simulink model "Expriment_All2"  (R2014a)
settings: Solver=FixedStepDiscrete  SolverMode=SingleTasking  StartTime=0.0  StopTime=inf  FixedStep=0.01  RelTol=1e-3
PostLoadFcn:
  | h_RPStest = RPStest;
model workspace (MAT data in the model file):
  gtest = 0
undefined symbols (not defined in the file or in its folder): avert, avert_freq_factor, avert_gaze_dirs_chance, avert_gaze_duration_factor, avert_head_frequency_factor, avert_head_speed, BML, BML1, BML2, bmlsL, bmlsM, bodyBusyFlag, clock, emotion_amount_factor, faceBusyFlag, fileID, GAZE_WIN, gazing, mut_freq_factor, mutual_gaze_duration_factor, P, pose_cat_chance, pose_chanc_factor, pose_chance_factor, pose_frequency_factor, pose_lean, pose_lean_flag, pose_speed, pose_twitch, pr, serial, STATE_BEFORE, STATE_GO, STATE_OVER, STATE_READY, Stateflow
libraries: simulink x24, instrumentlib x6, lib_affectiveChar_behavior x2, realtime_pacer_lib x2, lib_affectiveChar_input x1
(part 7 of 7)

== stateflow chart Expriment_All2/CharacterControl/Gaze_Controller ==
  note: ?
  note: ?
  note: implement PERSONALITY-based gaze behavior: ( setAffectFactors function)
      | HEHN:mutual dur more,head avert freq more,high freq of change btw mut/avert
      | LEHN:avert dur  more,head avert freq more, high freq of change btw mut/avert
      | HELN:mutual dur  more,head avert freq more,high freq of change btw mut/avert
      | LELN:avert  dur more,head avert freq more,high freq of change btw mut/avert
  note: ?
  note: implement emotion-based gaze behavior, Valence/Arousal: ref?(setAffectFactors)
      | V+A+ (excite,happy):high mutual dur,head avert freq less,high freq of change btw mut/avert
      | V-A+ (fear,frust): mid mut/avert,,head avert freq mid,high freq of change btw mut/avert
      | V+A- (idle, calm): mid mut/avert,head avert freq mid,low freq of change btw mut/avert
      | V-A- (bored,sad):  avert dur more,,head avert freq more,,high freq of change btw mut/avert
  note: Idle gaze impelementation:
      | For chanceO instead of range btw 5,15 we pick 3,15; 3,8 for eye due to Smartbody gaze DOF(5', 12') and 9 to 15 for head
      | A=saccade magnitude
      | CHANCEO=P=chance of occure (random num btw 0 and 15)  -> for us:3 to 8
      | magnitude=A=-6.9 * log(P/15.7), A is a value btw 0 and 27 ->for us: 5 to 12
      | Eye Alives' Image 5
      | -Saccade direction: Up/Down/Left/Right/UL/UR/DL/DR
      | 15% chance of pures and 8% chance of others.
      | -Duration D=D0+d*A-> avertDur=(25+2.5*magnitude)->36 to 52
      | d=2.4 msec/degree;  D0=25
      | For more info check Badler's Eye's Alive paper
  note: Idle gaze impelementation cont.:
      |
      | mut=Percent chance of stay in mutual gaze based on time is mut=[0.0003 -0.18 32]  %chance of no change from mutual =Y=0.0003x2 - 0.18 x +32
      | polyval(mut,t) %  t btw 1 to 400, mut btw 30 and 4
      |
      | avert=Percent chance of stay in avert gaze based on time:   avert=[-0.0034 0.23 -6.7 79]
      | polyval(avert,t)  % t btw 0 and 60 , avert btw 79 and -100?!
      | Eye's Alive paper's image 7
  note: avert_head_frequency_factor:
      | Riggio suggested that extraverts have a higher head movement frequency than introverts.
      | Riggio, R., Friedman, H. 1986. Impression formation: The role of expressive behavior. In Journal of Personality and Social Psychology 50(2), 421-427
  note: impelemnt attention:
      | all gaze movements are based on gazeTarget pawn in smartbody. Idle gaze stops when agent attends something since it gazes that. If user starts moving the idle gaze stops.It also stops in RPS game,ready and go states.
  note: Extroverts maintain eye-contact for longer.
      | Mehrabian, A. 1969. Significance of posture and position in
      | the communication of attitude and status relationships. In
      | Psychological Bulletin 71(5), 359-372.
  note: Note on modulization of affect (personality/emotion): I could have a seperate module for affect impact on all behaviors (gaze/pose/face). But I see the personality not as a seperate module but as a factor on (or layer on top of) eachbehavior. That's why I defined a matlab function (affect) in which emotion/personality facors affects different parameters of each behavior inside that behavior module. But for modulization, I also specify 0 as no personality in case someone don't want to use it.
  state headAvert [parallel]
    settings: executionOrder=2
    state stateInit1
      entry: STATE_OVER=3;STATE_BEFORE=4;STATE_READY=7;STATE_GO=1; gameState=14;
      GAZE_GUI=1;GAZE_SOFTEYE=2;GAZE_USER_HAND=3;GAZE_WIN=4;
      n=encStr2Arr(' ');bmlsL=[n n n n n];newBmlsL=[n n n n n];
      avert_head_speed=1;avertH=0;
    state stateRandGen1
      entry:
      gazeUserHandChance=randArray(:,4);gazeGUIChance=randArray(:,5);
      randHeadDur=((25+2.5*magnitude)*avert_gaze_duration_factor)/3;
    state stateHeadNeutralN1
      entry: [P,BMLl]= idleNormalHeadTable(12);
      newBmlsL=insertQueueLow(bmlsL,BMLl); bmlsL=newBmlsL;
      avertH=0;
    state stateAvertHeadNormal
      entry: avert=1; [P,BMLl]= idleNormalHeadTable(randArray(:,18));
      newBmlsL=insertQueueLow(bmlsL,BMLl); bmlsL=newBmlsL;
    state stateHeadNeutralF1
      entry: [P,BMLl]= idleFastUpHeadTable(22) ;
      newBmlsL=insertQueueLow(bmlsL,BMLl); bmlsL=newBmlsL;
      avertH=0;
    state stateAvertHeadFast%btw(1,20)
      entry: avert=1; [P,BMLl]= idleFastUpHeadTable(randArray(:,18));
      newBmlsL=insertQueueLow(bmlsL,BMLl); bmlsL=newBmlsL;
      %disp(decArr2Str(BMLl));
    state stateHeadNeutralS1
      entry: [P,BMLl]= idleSlowDownHeadTable(19) ;
      newBmlsL=insertQueueLow(bmlsL,BMLl); bmlsL=newBmlsL;
      avertH=0;
    state stateAvertHeadSlow%btw(1,18)
      entry: avert=1; [P,BMLl]= idleSlowDownHeadTable(randArray(:,19));
      newBmlsL=insertQueueLow(bmlsL,BMLl); bmlsL=newBmlsL;
    state stateGazingGUI
      entry: [P,BMLl]=  idleGazeTable(22) ;
      newBmlsL=insertQueueLow(bmlsL,BMLl); bmlsL=newBmlsL;
    state stateGazingUserHand
      entry: [P,BMLl]= idleGazeTable(23);
      newBmlsL=insertQueueLow(bmlsL,BMLl); bmlsL=newBmlsL;
    (default) -> stateInit1
    stateInit1 -> stateRandGen1 : [avertH==1]
    stateRandGen1 -> stateRandGen1 [order 4] : after(floor(randHeadDur/5),secs)
    stateRandGen1 -> stateGazingUserHand [order 2] : [([gazeUserHandChance==1])&([gazing==GAZE_USER_HAND])]
    stateRandGen1 -> stateGazingGUI [order 3] : [([gazeGUIChance==1])&([gazing==GAZE_GUI])]
    stateRandGen1 -> (junction 539) [order 1] : [[bodyBusyFlag~=1]&[faceBusyFlag~=1]&[ gameState~= STATE_GO]&[ gameState~= STATE_READY]&[avertH==1]]
    stateHeadNeutralS1 -> stateRandGen1 : after(2,secs)
    stateHeadNeutralF1 -> stateRandGen1 : after(2,secs)
    stateHeadNeutralN1 -> stateRandGen1 : after(2,secs)
    (junction 539) -> stateAvertHeadNormal [order 2] : [avert_head_speed==1]
    (junction 539) -> stateAvertHeadFast%btw(1,20) [order 1] : [avert_head_speed==2]
    (junction 539) -> stateAvertHeadSlow%btw(1,18) [order 3] : [avert_head_speed==3]
    stateAvertHeadNormal -> stateHeadNeutralN1 : after(randHeadDur,secs)
    (junction 508) -> stateHeadNeutralN1 [order 2] : [avert_head_speed==1]
    stateAvertHeadFast%btw(1,20) -> stateHeadNeutralF1 : after(randHeadDur,secs)
    (junction 508) -> stateHeadNeutralF1 [order 1] : [avert_head_speed==2]
    stateAvertHeadSlow%btw(1,18) -> stateHeadNeutralS1 : after(randHeadDur+20,secs)
    (junction 508) -> stateHeadNeutralS1 [order 3] : [avert_head_speed==3]
    stateGazingGUI -> (junction 508) : after(10,secs)
    stateGazingUserHand -> (junction 508) : after(10,secs)
  state stateGazeIde [parallel]
    settings: executionOrder=1
    state setBlinkRate
      entry: str= blinkFunction(blinkperiod_min,blinkperiod_max) ;
      sendSBM(str);blink_flag=0;
    state stateInit
      entry: STATE_OVER=3;STATE_BEFORE=4;STATE_READY=7;STATE_GO=1; gameState=14;
      n=encStr2Arr(' ');bmlsL=[n n n n n];newBmlsL=[n n n n n];
      mutual_gaze_duration_factor=1;avert_gaze_duration_factor=1;avert_gaze_dirs_chance=0;
      avert_freq_factor=1;mut_freq_factor=1;avert_head_frequency_factor=20;
      avert=1;avertH=0;currentTime=1;
      blink_flag=0;blinkperiod_min=5;blinkperiod_max=9;
    note: if already mutual do not send mut bml.
    state mutAgain
      entry:chanceO=randArray(:,17);
      magnitude=-6.9*log(chanceO/15.7);
      mutDur=((25+2.5*magnitude)*mutual_gaze_duration_factor)/7;
    state stateCheckMutCont
      entry:  coder.extrinsic('get_param');
      currentTime=get_param('Expriment_All','SimulationTime');
      mutContF=[0.0003 -0.18 32];
      CHANCEM=randArray(:,6);%btw 0,100
      mutContChance=polyval(mutContF,currentTime);
      mutContChance=mutContChance*mut_freq_factor;
    state stateAvert
      entry:%btw 1,100
      randHeadChance=randArray(:,3);
    state stateAvertEye
      entry:  avert=1;
      chanceO=randArray(:,7);%btw 3,8
      magnitude=-6.9*log(chanceO/15.7);
      avertDur=((25+2.5*magnitude)*avert_gaze_duration_factor)/7;
      gazeDir=randArray(:,8);
      BMLl= idleGazeFunction(gazeDir,floor(magnitude),avert_gaze_dirs_chance) ;
      newBmlsL=insertQueueLow(bmlsL,BMLl);
      bmlsL=newBmlsL;%fprintf(',A:'); fprintf('%1.1f',avertDur);
    state stateAvertHead
      entry:avertH=1;
      chanceH=randArray(:,25);%btw 8,15
      magnitude=-6.9*log(chanceH/15.7);
      avertDur=((25+2.5*magnitude)*avert_gaze_duration_factor)/7;
      gazeDir=randArray(:,8);
    state stateMutualGazeE
      entry:chanceO=randArray(:,17);%btw 3,8
      magnitude=-6.9*log(chanceO/15.7);
      mutDur=((25+2.5*magnitude)*mutual_gaze_duration_factor)/7;
      [P,BMLl]= idleNormalHeadTable(11) ;%neutralGaze
      avert=0;
      newBmlsL=insertQueueLow(bmlsL,BMLl);
      bmlsL=newBmlsL;%fprintf(',M:'); fprintf('%1.1f',mutDur);
    state stateCheckAvertCont
      entry:
      coder.extrinsic('get_param');
      currentTime=get_param('Expriment_All','SimulationTime');
      %avertContF=[-0.0034 0.23 -6.7 79];
      avertContF=[0.0003 -0.18 32];
      avertContChance=polyval(avertContF,currentTime);
      avertContChance=avertContChance*avert_freq_factor;
      CHANCEA=randArray(:,9);%btw 0,100
    setBlinkRate -> stateAvert [order 2]
    stateAvert -> setBlinkRate [order 1] : [blink_flag==1]%order first
    stateCheckMutCont -> setBlinkRate [order 1] : [blink_flag==1]%order first
    setBlinkRate -> stateCheckMutCont [order 1] : after(5,secs)
    (default) -> stateInit
    stateInit -> stateCheckMutCont : [[bodyBusyFlag~=1]&[faceBusyFlag~=1]&[ gameState~= STATE_GO]&[ gameState~= STATE_READY]]
    mutAgain -> stateCheckMutCont : after(floor(mutDur),secs)
    stateCheckMutCont -> mutAgain [order 4] : [avert==0]%order after avert 1
    stateAvert -> (junction 577) [order 2]
    (junction 577) -> stateAvertEye [order 1] : [avert_head_frequency_factor<=randHeadChance]
    (junction 577) -> stateAvertHead [order 2] : [avert_head_frequency_factor>randHeadChance]
    stateCheckMutCont -> stateAvert [order 2] : [[CHANCEM>mutContChance]&[bodyBusyFlag~=1]&[faceBusyFlag~=1]&[ gameState~= STATE_GO]&[ gameState~= STATE_READY]]
    (junction 200) -> stateAvert [order 2] : [[CHANCEA<=avertContChance]&[ gameState~= STATE_GO]&[ gameState~= STATE_READY]]
    stateCheckMutCont -> (junction 323) [order 3] : [[avert==1]&[CHANCEM<=mutContChance]&[bodyBusyFlag~=1]&[faceBusyFlag~=1]&[ gameState~= STATE_GO]&[ gameState~= STATE_READY]]
    stateMutualGazeE -> stateCheckMutCont : after(floor(mutDur),secs)
    stateAvertHead -> (junction 588) : [avertH==0]
    stateAvertEye -> (junction 581) : after(floor(avertDur),secs)
    (junction 588) -> (junction 581) : after(5,secs)
    (junction 581) -> stateCheckAvertCont
    stateCheckAvertCont -> (junction 200)
    (junction 200) -> (junction 323) [order 1] : [[avertH==0]&[CHANCEA>avertContChance]&[ gameState~= STATE_GO]&[ gameState~= STATE_READY]]
    (junction 323) -> stateMutualGazeE
  note: idleGaze(1,8) used for gaze,
      | idleGaze(9,16) used for head,
      | idleGaze(17) used for neutralHead
      | idleGaze(18) used for gaze at board
  note: The result of facial expr module showed that if we only consider emotion on facial expr generation, it leads to non-consistent behavior because emotion also affects how we gaze, pose and gesture. If your face shows boredom but there is no evidence in other parts of the body it looks not consistent.
      | But the question is how much of these behaviors are affected by personality and how much with emotion. e.g. highly extroverts seems to mutual gaze more, is it because they generally experience more positive valence. or neurotics avert more is it becasue of high arousal?
  state sendSBM(In) [function]
  data: p function_output double size=1; bmlID function_input double; gazeBML function_output double size=[1000,1]; p function_output double size=1; bmlID function_input double; gazeBML function_output double size=[1000,1]; p function_output double size=1; bmlID function_input double; gazeBML function_output double size=[1000,1]; p function_output double size=1; bmlID function_input double; gazeBML function_output double size=[1000,1]; p function_output double size=1; bmlID function_input double size=1; gazeBML function_output double size=[1000,1]; p function_output double size=1; bmlID function_input double; gazeBML function_output double size=[1000,1]; dir function_input double size=1; mag function_input double size=1; arrBML function_output double size=[1000,1]; p function_output double size=1; bmlID function_input double; poseBML function_output double size=[1000,1]; dir function_input double size=1; mag function_input double size=1; arrBML function_output double size=[1000,1]; dirChance function_input double size=1; headSpeed function_input double size=1; dir function_input double size=1; mag function_input double size=1; arrBML function_output double size=[1000,1]; dirChance function_input double size=1; bmls function_input double size=[1000,5]; myBML function_input double size=[1000,1]; newBmls function_output double size=[1000,5]; blinkPeriodMin function_input double size=1; arrSBM function_output double size=[1000,1]; blinkPeriodMax function_input double size=1; In function_input double size=[1000 1]; boredom data_store_memory size=2; BOREDOM_THRESHOLD data_store_memory size=2; randAvertGazeChance data_store_memory size=2; randPoseChance data_store_memory size=2; interest data_store_memory size=2; randGazeDur data_store_memory size=2; gazing data_store_memory size=2; GAZE_SOFTEYE data_store_memory size=2; GAZE_GUI data_store_memory size=2; GAZE_USER_HAND data_store_memory size=2; GAZE_WIN data_store_memory size=2; randHeadDur local; randHeadDurOver local; gameState output double size=1; avert data_store_memory size=2; STATE_BEFORE data_store_memory size=2; STATE_OVER data_store_memory size=2; STATE_READY data_store_memory size=2; avertContChance local; gazeGUIChance local; mutContChance local; mutContF local; CHANCEM local; avertDur local; gazeDir local; CHANCEA local; magnitude local; randHeadChance local; avertContF local; gazeUserHandChance local; bmlsL data_store_memory size=[256,1]; pr data_store_memory; P data_store_memory; chanceO local; fileID data_store_memory; STATE_GO data_store_memory; bodyBusyFlag data_store_memory; BMLl local double size=[1000,1]; BML data_store_memory size=[256,1]; newBmlsL local double size=[1000,5]; n local; randArray input double size=[1,40]; mutDur local; personality input double size=1; mF local; hF local; aF local; avertH data_store_memory; inV input double size=1; inA input size=1; mFe local; hFe local; aFe local; personalityChange input boolean size=1; faceBusyFlag data_store_memory; gazeArray input double size=[1,6]; avert_gaze_dirs_chance data_store_memory; avert_head_speed data_store_memory; avert_head_frequency_factor data_store_memory; avert_gaze_duration_factor data_store_memory; mutual_gaze_duration_factor data_store_memory; chanceH local; currentTime local; avert_freq_factor data_store_memory; mut_freq_factor data_store_memory; blink_flag data_store_memory; blinkperiod_min data_store_memory; str local; blinkperiod_max data_store_memory
  events: secs input RISING_EDGE_EVENT
  function [p,gazeBML]=idleSlowDownHeadTable(bmlID):
    | function [p,gazeBML]=idleSlowDownHeadTable(bmlID)
    | 
    | aVarTruthTableCondition_1 = false;
    | aVarTruthTableCondition_2 = false;
    | aVarTruthTableCondition_3 = false;
    | aVarTruthTableCondition_4 = false;
    | aVarTruthTableCondition_5 = false;
    | aVarTruthTableCondition_6 = false;
    | aVarTruthTableCondition_7 = false;
    | aVarTruthTableCondition_8 = false;
    | aVarTruthTableCondition_9 = false;
    | aVarTruthTableCondition_10 = false;
    | aVarTruthTableCondition_11 = false;
    | aVarTruthTableCondition_12 = false;
    | aVarTruthTableCondition_13 = false;
    | aVarTruthTableCondition_14 = false;
    | aVarTruthTableCondition_15 = false;
    | aVarTruthTableCondition_16 = false;
    | aVarTruthTableCondition_17 = false;
    | aVarTruthTableCondition_18 = false;
    | aVarTruthTableCondition_19 = false;
    | 
    | 
    | 
    | aVarTruthTableCondition_1 = logical(bmlID==1);
    | 
    | 
    | aVarTruthTableCondition_2 = logical(bmlID==2);
    | 
    | 
    | aVarTruthTableCondition_3 = logical(bmlID==3);
    | 
    | 
    | aVarTruthTableCondition_4 = logical(bmlID==4);
    | 
    | 
    | aVarTruthTableCondition_5 = logical(bmlID==5);
    | 
    | 
    | aVarTruthTableCondition_6 = logical(bmlID==6);
    | 
    | 
    | aVarTruthTableCondition_7 = logical(bmlID==7);
    | 
    | 
    | aVarTruthTableCondition_8 = logical(bmlID==8);
    | 
    | 
    | aVarTruthTableCondition_9 = logical(bmlID==9);
    | 
    | 
    | aVarTruthTableCondition_10 = logical(bmlID==10);
    | 
    | 
    | aVarTruthTableCondition_11 = logical(bmlID==11);
    | 
    | 
    | aVarTruthTableCondition_12 = logical(bmlID==12);
    | 
    | 
    | aVarTruthTableCondition_13 = logical(bmlID==13);
    | 
    | 
    | aVarTruthTableCondition_14 = logical(bmlID==14);
    | 
    | 
    | aVarTruthTableCondition_15 = logical(bmlID==15);
    | 
    | 
    | aVarTruthTableCondition_16 = logical(bmlID==16);
    | 
    | 
    | aVarTruthTableCondition_17 = logical(bmlID==17);
    | 
    | 
    | aVarTruthTableCondition_18 = logical(bmlID==18);
    | 
    | 
    | aVarTruthTableCondition_19 = logical(bmlID==19);
    | 
    | if (aVarTruthTableCondition_1)
    |     aFcnTruthTableAction_1();
    | elseif (aVarTruthTableCondition_2)
    |     aFcnTruthTableAction_2();
    | elseif (aVarTruthTableCondition_3)
    |     aFcnTruthTableAction_3();
    | elseif (aVarTruthTableCondition_4)
    |     aFcnTruthTableAction_4();
    | elseif (aVarTruthTableCondition_5)
    |     aFcnTruthTableAction_1();
    | elseif (aVarTruthTableCondition_6)
    |     aFcnTruthTableAction_2();
    | elseif (aVarTruthTableCondition_7)
    |     aFcnTruthTableAction_3();
    | elseif (aVarTruthTableCondition_8)
    |     aFcnTruthTableAction_4();
    | elseif (aVarTruthTableCondition_9)
    |     aFcnTruthTableAction_5();
    | elseif (aVarTruthTableCondition_10)
    |     aFcnTruthTableAction_6();
    | elseif (aVarTruthTableCondition_11)
    |     aFcnTruthTableAction_7();
    | elseif (aVarTruthTableCondition_12)
    |     aFcnTruthTableAction_8();
    | elseif (aVarTruthTableCondition_13)
    |     aFcnTruthTableAction_9();
    | elseif (aVarTruthTableCondition_14)
    |     aFcnTruthTableAction_10();
    | elseif (aVarTruthTableCondition_15)
    |     aFcnTruthTableAction_11();
    | elseif (aVarTruthTableCondition_16)
    |     aFcnTruthTableAction_12();
    | elseif (aVarTruthTableCondition_17)
    |     aFcnTruthTableAction_13();
    | elseif (aVarTruthTableCondition_18)
    |     aFcnTruthTableAction_14();
    | elseif (aVarTruthTableCondition_19)
    |     aFcnTruthTableAction_15();
    | else % Default
    |     aFcnTruthTableAction_1();
    | end
    | 
    | function aFcnTruthTableAction_1()
    | 
    | % DownleftHeadSlow1
    | 
    | gazeBML=encStr2Arr('<?xml version="1.0" ?><act><bml><gaze direction="DOWNLEFT" angle="15" sbm:joint-range="EYES NECK" sbm:time-hint="1.2" target="gazeTarget"/></bml></act>');p=3;
    | 
    | function aFcnTruthTableAction_2()
    | 
    | % DownleftHeadSlow2
    | 
    | gazeBML=encStr2Arr('<?xml version="1.0" ?><act><bml><gaze direction="DOWNLEFT" angle="20" sbm:joint-range="EYES NECK" sbm:time-hint="1.2" target="gazeTarget"/></bml></act>');p=3;
    | 
    | function aFcnTruthTableAction_3()
    | 
    | % DownleftHeadSlow3
    | 
    | gazeBML=encStr2Arr('<?xml version="1.0" ?><act><bml><gaze direction="DOWNLEFT" angle="25" sbm:joint-range="EYES NECK" sbm:time-hint="1.2" target="gazeTarget"/></bml></act>');p=3;
    | 
    | function aFcnTruthTableAction_4()
    | 
    | % DownleftHeadSlow4
    | 
    | gazeBML=encStr2Arr('<?xml version="1.0" ?><act><bml><gaze direction="DOWNLEFT" angle="30" sbm:joint-range="EYES NECK" sbm:time-hint="1.2" target="gazeTarget"/></bml></act>');p=3;
    | 
    | function aFcnTruthTableAction_5()
    | 
    | % DownrightHeadSlow1
    | 
    | gazeBML=encStr2Arr('<?xml version="1.0" ?><act><bml><gaze direction="DOWNRIGHT" angle="15" sbm:joint-range="EYES NECK" sbm:time-hint="1.2" target="gazeTarget"/></bml></act>');p=3;
    | 
    | function aFcnTruthTableAction_6()
    | 
    | % DownrightHeadSlow2
    | 
    | gazeBML=encStr2Arr('<?xml version="1.0" ?><act><bml><gaze direction="DOWNRIGHT" angle="20" sbm:joint-range="EYES NECK" sbm:time-hint="1.2" target="gazeTarget"/></bml></act>');p=3;
    | 
    | function aFcnTruthTableAction_7()
    | 
    | % DownrightHeadSlow3
    | 
    | gazeBML=encStr2Arr('<?xml version="1.0" ?><act><bml><gaze direction="DOWNRIGHT" angle="25" sbm:joint-range="EYES NECK" sbm:time-hint="1.2" target="gazeTarget"/></bml></act>');p=3;
    | 
    | function aFcnTruthTableAction_8()
    | 
    | % DownrightHeadSlow4
    | 
    | gazeBML=encStr2Arr('<?xml version="1.0" ?><act><bml><gaze direction="DOWNRIGHT" angle="30" sbm:joint-range="EYES NECK" sbm:time-hint="1.2" target="gazeTarget"/></bml></act>');p=3;
    | 
    | function aFcnTruthTableAction_9()
    | 
    | % DownHeadSlow1
    | 
    | gazeBML=encStr2Arr('<?xml version="1.0" ?><act><bml><gaze direction="DOWN" angle="15" sbm:joint-range="EYES NECK" sbm:time-hint="1.2" target="gazeTarget"/></bml></act>');p=3;
    | 
    | function aFcnTruthTableAction_10()
    | 
    | % DownHeadSlow2
    | 
    | gazeBML=encStr2Arr('<?xml version="1.0" ?><act><bml><gaze direction="DOWN" angle="20" sbm:joint-range="EYES NECK" sbm:time-hint="1.2" target="gazeTarget"/></bml></act>');p=3;
    | 
    | function aFcnTruthTableAction_11()
    | 
    | % DownHeadSlow3
    | 
    | gazeBML=encStr2Arr('<?xml version="1.0" ?><act><bml><gaze direction="DOWN" angle="25" sbm:joint-range="EYES NECK" sbm:time-hint="1.2" target="gazeTarget"/></bml></act>');p=3;
    | 
    | function aFcnTruthTableAction_12()
    | 
    | % DownHeadSlow4
    | 
    | gazeBML=encStr2Arr('<?xml version="1.0" ?><act><bml><gaze direction="DOWN" angle="30" sbm:joint-range="EYES NECK" sbm:time-hint="1.2" target="gazeTarget"/></bml></act>');p=3;
    | 
    | function aFcnTruthTableAction_13()
    | 
    | % LEFTHeadDSlow
    | 
    | gazeBML=encStr2Arr('<?xml version="1.0" ?><act><bml><gaze direction="DOWNLEFT" angle="10" sbm:joint-range="EYES NECK" sbm:time-hint="1.2" target="gazeTarget"/></bml></act>');p=3;
    | 
    | function aFcnTruthTableAction_14()
    | 
    | % RightHeadDSlow
    | 
    | gazeBML=encStr2Arr('<?xml version="1.0" ?><act><bml><gaze direction="DOWNRIGHT" angle="10" sbm:joint-range="EYES NECK" sbm:time-hint="1.2" target="gazeTarget"/></bml></act>');p=3;
    | 
    | function aFcnTruthTableAction_15()
    | 
    | % introvertHeadNeutral
    | 
    | gazeBML=encStr2Arr('<?xml version="1.0" ?><act><bml><gaze angle="5" direction="DOWN" sbm:joint-range="EYES BACK" sbm:time-hint="1.2" target="gazeTarget"/></bml></act>'); p=3;
  function [p,gazeBML]=idleGazeTable(bmlID):
    | function [p,gazeBML]=idleGazeTable(bmlID)
    | 
    | aVarTruthTableCondition_1 = false;
    | aVarTruthTableCondition_2 = false;
    | aVarTruthTableCondition_3 = false;
    | aVarTruthTableCondition_4 = false;
    | aVarTruthTableCondition_5 = false;
    | aVarTruthTableCondition_6 = false;
    | aVarTruthTableCondition_7 = false;
    | aVarTruthTableCondition_8 = false;
    | aVarTruthTableCondition_9 = false;
    | aVarTruthTableCondition_10 = false;
    | aVarTruthTableCondition_11 = false;
    | aVarTruthTableCondition_12 = false;
    | aVarTruthTableCondition_13 = false;
    | aVarTruthTableCondition_14 = false;
    | aVarTruthTableCondition_15 = false;
    | aVarTruthTableCondition_16 = false;
    | aVarTruthTableCondition_17 = false;
    | aVarTruthTableCondition_18 = false;
    | aVarTruthTableCondition_19 = false;
    | aVarTruthTableCondition_20 = false;
    | aVarTruthTableCondition_21 = false;
    | aVarTruthTableCondition_22 = false;
    | aVarTruthTableCondition_23 = false;
    | 
    | 
    | 
    | aVarTruthTableCondition_1 = logical(bmlID==1);
    | 
    | 
    | aVarTruthTableCondition_2 = logical(bmlID==2);
    | 
    | 
    | aVarTruthTableCondition_3 = logical(bmlID==3);
    | 
    | 
    | aVarTruthTableCondition_4 = logical(bmlID==4);
    | 
    | 
    | aVarTruthTableCondition_5 = logical(bmlID==5);
    | 
    | 
    | aVarTruthTableCondition_6 = logical(bmlID==6);
    | 
    | 
    | aVarTruthTableCondition_7 = logical(bmlID==7);
    | 
    | 
    | aVarTruthTableCondition_8 = logical(bmlID==8);
    | 
    | 
    | aVarTruthTableCondition_9 = logical(bmlID==9);
    | 
    | 
    | aVarTruthTableCondition_10 = logical(bmlID==10);
    | 
    | 
    | aVarTruthTableCondition_11 = logical(bmlID==11);
    | 
    | 
    | aVarTruthTableCondition_12 = logical(bmlID==12);
    | 
    | 
    | aVarTruthTableCondition_13 = logical(bmlID==13);
    | 
    | 
    | aVarTruthTableCondition_14 = logical(bmlID==14);
    | 
    | 
    | aVarTruthTableCondition_15 = logical(bmlID==15);
    | 
    | 
    | aVarTruthTableCondition_16 = logical(bmlID==16);
    | 
    | % neutralHead
    | 
    | aVarTruthTableCondition_17 = logical(bmlID==17);
    | 
    | % gazeAtGUIRachel
    | 
    | aVarTruthTableCondition_18 = logical(bmlID==18);
    | 
    | % softeye
    | 
    | aVarTruthTableCondition_19 = logical(bmlID==19);
    | 
    | % softeyebrow
    | 
    | aVarTruthTableCondition_20 = logical(bmlID==20);
    | 
    | % gazeUserHand
    | 
    | aVarTruthTableCondition_21 = logical(bmlID==21);
    | 
    | % gazeGUIBrad
    | 
    | aVarTruthTableCondition_22 = logical(bmlID==22);
    | 
    | % gazeHandBrad
    | 
    | aVarTruthTableCondition_23 = logical(bmlID==23);
    | 
    | if (aVarTruthTableCondition_1)
    |     aFcnTruthTableAction_1();
    | elseif (aVarTruthTableCondition_2)
    |     aFcnTruthTableAction_2();
    | elseif (aVarTruthTableCondition_3)
    |     aFcnTruthTableAction_3();
    | elseif (aVarTruthTableCondition_4)
    |     aFcnTruthTableAction_4();
    | elseif (aVarTruthTableCondition_5)
    |     aFcnTruthTableAction_5();
    | elseif (aVarTruthTableCondition_6)
    |     aFcnTruthTableAction_6();
    | elseif (aVarTruthTableCondition_7)
    |     aFcnTruthTableAction_7();
    | elseif (aVarTruthTableCondition_8)
    |     aFcnTruthTableAction_8();
    | elseif (aVarTruthTableCondition_9)
    |     aFcnTruthTableAction_9();
    | elseif (aVarTruthTableCondition_10)
    |     aFcnTruthTableAction_10();
    | elseif (aVarTruthTableCondition_11)
    |     aFcnTruthTableAction_11();
    | elseif (aVarTruthTableCondition_12)
    |     aFcnTruthTableAction_12();
    | elseif (aVarTruthTableCondition_13)
    |     aFcnTruthTableAction_13();
    | elseif (aVarTruthTableCondition_14)
    |     aFcnTruthTableAction_14();
    | elseif (aVarTruthTableCondition_15)
    |     aFcnTruthTableAction_15();
    | elseif (aVarTruthTableCondition_16)
    |     aFcnTruthTableAction_16();
    | elseif (aVarTruthTableCondition_17)
    |     aFcnTruthTableAction_17();
    | elseif (aVarTruthTableCondition_18)
    |     aFcnTruthTableAction_18();
    | elseif (aVarTruthTableCondition_19)
    |     aFcnTruthTableAction_19();
    | elseif (aVarTruthTableCondition_20)
    |     aFcnTruthTableAction_20();
    | elseif (aVarTruthTableCondition_21)
    |     aFcnTruthTableAction_21();
    | elseif (aVarTruthTableCondition_22)
    |     aFcnTruthTableAction_22();
    | elseif (aVarTruthTableCondition_23)
    |     aFcnTruthTableAction_23();
    | else % Default
    |     aFcnTruthTableAction_1();
    | end
    | 
    | function aFcnTruthTableAction_1()
    | 
    | % LeftS
    | 
    | gazeBML=encStr2Arr('<?xml version="1.0" ?><act><bml><gaze angle="12" direction="LEFT" sbm:joint-range="EYES" target="gazeTarget"/></bml></act>');p=3;
    | 
    | function aFcnTruthTableAction_2()
    | 
    | % RightS
    | 
    | gazeBML=encStr2Arr('<?xml version="1.0" ?><act><bml><gaze angle="12" direction="RIGHT" sbm:joint-range="EYES" target="gazeTarget"/></bml></act>');p=3;
    | 
    | function aFcnTruthTableAction_3()
    | 
    | % UpS
    | 
    | gazeBML=encStr2Arr('<?xml version="1.0" ?><act><bml><gaze angle="12" direction="UP" sbm:joint-range="EYES" target="gazeTarget"/></bml></act>');p=3;
    | 
    | function aFcnTruthTableAction_4()
    | 
    | % DownS
    | 
    | gazeBML=encStr2Arr('<?xml version="1.0" ?><act><bml><gaze angle="12" direction="DOWN" sbm:joint-range="EYES" target="gazeTarget"/></bml></act>');p=3;
    | 
    | function aFcnTruthTableAction_5()
    | 
    | % UpLeftS
    | 
    | gazeBML=encStr2Arr('<?xml version="1.0" ?><act><bml><gaze angle="12" direction="UPLEFT" sbm:joint-range="EYES" target="gazeTarget"/></bml></act>');p=3;
    | 
    | function aFcnTruthTableAction_6()
    | 
    | % UpRightS
    | 
    | gazeBML=encStr2Arr('<?xml version="1.0" ?><act><bml><gaze angle="12" direction="UPRIGHT" sbm:joint-range="EYES" target="gazeTarget"/></bml></act>');p=3;
    | 
    | function aFcnTruthTableAction_7()
    | 
    | % DownLeftS
    | 
    | gazeBML=encStr2Arr('<?xml version="1.0" ?><act><bml><gaze angle="12" direction="DOWNLEFT" sbm:joint-range="EYES" target="gazeTarget"/></bml></act>');p=3;
    | 
    | function aFcnTruthTableAction_8()
    | 
    | % DownRightS
    | 
    | gazeBML=encStr2Arr('<?xml version="1.0" ?><act><bml><gaze angle="12" direction="DOWNRIGHT" sbm:joint-range="EYES" target="gazeTarget"/></bml></act>');p=3;
    | 
    | function aFcnTruthTableAction_9()
    | 
    | % Downleft
    | 
    | gazeBML=encStr2Arr('<?xml version="1.0" ?><act><bml><gaze direction="DOWNLEFT" angle="15" sbm:joint-range="EYES NECK" sbm:time-hint="1" target="gazeTarget"/></bml></act>');p=3;
    | 
    | function aFcnTruthTableAction_10()
    | 
    | % Downright
    | 
    | gazeBML=encStr2Arr('<?xml version="1.0" ?><act><bml><gaze direction="DOWNRIGHT" angle="15" sbm:joint-range="EYES NECK" sbm:time-hint="1" target="gazeTarget"/></bml></act>');p=3;
    | 
    | function aFcnTruthTableAction_11()
    | 
    | % Down
    | 
    | gazeBML=encStr2Arr('<?xml version="1.0" ?><act><bml><gaze direction="DOWN" angle="15" sbm:joint-range="EYES NECK" sbm:time-hint="1" target="gazeTarget"/></bml></act>');p=3;
    | 
    | function aFcnTruthTableAction_12()
    | 
    | % Upright
    | 
    | gazeBML=encStr2Arr('<?xml version="1.0" ?><act><bml><gaze direction="UPRIGHT" angle="15" sbm:joint-range="EYES NECK" sbm:time-hint="1" target="gazeTarget"/></bml></act>');p=3;
    | 
    | function aFcnTruthTableAction_13()
    | 
    | % Upleft
    | 
    | gazeBML=encStr2Arr('<?xml version="1.0" ?><act><bml><gaze direction="UPLEFT" angle="15" sbm:joint-range="EYES NECK" sbm:time-hint="1" target="gazeTarget"/></bml></act>');p=3;
    | 
    | function aFcnTruthTableAction_14()
    | 
    | % Up
    | 
    | gazeBML=encStr2Arr('<?xml version="1.0" ?><act><bml><gaze direction="UP" angle="15" sbm:joint-range="EYES NECK" sbm:time-hint="1" target="gazeTarget"/><gaze angle="10" direction="UP" sbm:joint-range="EYES" target="camera"/></bml></act>');p=3;
    | 
    | function aFcnTruthTableAction_15()
    | 
    | % Right
    | 
    | gazeBML=encStr2Arr('<?xml version="1.0" ?><act><bml><gaze direction="RIGHT" angle="15" sbm:joint-range="EYES NECK" sbm:time-hint="1" target="gazeTarget"/></bml></act>');p=3;
    | 
    | function aFcnTruthTableAction_16()
    | 
    | % LEFT
    | 
    | gazeBML=encStr2Arr('<?xml version="1.0" ?><act><bml><gaze direction="LEFT" angle="15" sbm:joint-range="EYES NECK" sbm:time-hint="1" target="gazeTarget"/></bml></act>');p=3;
    | 
    | function aFcnTruthTableAction_17()
    | 
    | % neutralHeadGaze
    | 
    | gazeBML=encStr2Arr('<?xml version="1.0" ?><act><bml><gaze target="gazeTarget" sbm:joint-range="EYES NECK" sbm:time-hint="1"/></bml></act>');p=3;
    | 
    | function aFcnTruthTableAction_18()
    | 
    | % gazeAtGUI
    | 
    | gazeBML=encStr2Arr('<?xml version="1.0" ?><act><bml><gaze angle="35" direction="DOWNRIGHT" sbm:joint-range="EYES" sbm:time-hint="0.2" target="gazeTarget"/><gaze angle="20" direction="RIGHT" sbm:joint-range="NECK" sbm:time-hint="0.3" target="camera"/></bml></act>');p=3;
    | 
    | function aFcnTruthTableAction_19()
    | 
    | % softeye
    | 
    | gazeBML=encStr2Arr('<?xml version="1.0" ?><act><bml><face amount="0.1" au="45" side="BOTH" type="facs"  start="0" ready="5" stroke="10" relax="15" end="20"  /></bml></act>');p=3;
    | 
    | function aFcnTruthTableAction_20()
    | 
    | % softeyebrow
    | 
    | gazeBML=encStr2Arr('<?xml version="1.0" ?><act><bml><face amount="0.5" au="1" side="BOTH" type="facs" start="0" ready="5" stroke="10" relax="15" end="20" /><face amount="0.5" au="2" side="BOTH" type="facs" start="0" ready="5" stroke="10" relax="15" end="20"/></bml></act>');p=3;
    | 
    | function aFcnTruthTableAction_21()
    | 
    | % gazeUserHand
    | 
    | gazeBML=encStr2Arr('<?xml version="1.0" ?><act><bml><gaze angle="-5" direction="POLAR" sbm:joint-range="EYES" sbm:time-hint="0.29" target="camera"/></bml></act>');p=3;
    | 
    | function aFcnTruthTableAction_22()
    | 
    | % gazeAtGUIBrad
    | 
    | gazeBML=encStr2Arr('<?xml version="1.0" ?><act><bml><gaze angle="30" direction="DOWNRIGHT" sbm:joint-range="EYES" sbm:time-hint="1.5" target="gazeTarget"/><gaze angle="15" direction="RIGHT" sbm:joint-range="NECK" sbm:time-hint="0.3" target="camera"/></bml></act>');p=2;
    | 
    | function aFcnTruthTableAction_23()
    | 
    | % gazeUserHandBrad
    | 
    | gazeBML=encStr2Arr('<?xml version="1.0" ?><act><bml><gaze angle="10" direction="DOWN" sbm:joint-range="EYES" sbm:time-hint="1.5" target="gazeTarget"/></bml></act>');p=2;
    | 
    | function aFcnTruthTableAction_24()
    | 
    | % blinkOnce
    | 
    | gazeBML=encStr2Arr('<?xml version="1.0" ?><act><bml><face type="FACS" side="BOTH" au="45" start="0" end="0.1" amount="1" /></bml></act>');p=3;
  function [p,gazeBML]=idleNormalHeadTable(bmlID):
    | function [p,gazeBML]=idleNormalHeadTable(bmlID)
    | 
    | aVarTruthTableCondition_1 = false;
    | aVarTruthTableCondition_2 = false;
    | aVarTruthTableCondition_3 = false;
    | aVarTruthTableCondition_4 = false;
    | aVarTruthTableCondition_5 = false;
    | aVarTruthTableCondition_6 = false;
    | aVarTruthTableCondition_7 = false;
    | aVarTruthTableCondition_8 = false;
    | aVarTruthTableCondition_9 = false;
    | aVarTruthTableCondition_10 = false;
    | aVarTruthTableCondition_11 = false;
    | aVarTruthTableCondition_12 = false;
    | 
    | 
    | 
    | aVarTruthTableCondition_1 = logical(bmlID==1);
    | 
    | 
    | aVarTruthTableCondition_2 = logical(bmlID==2);
    | 
    | 
    | aVarTruthTableCondition_3 = logical(bmlID==3);
    | 
    | 
    | aVarTruthTableCondition_4 = logical(bmlID==4);
    | 
    | 
    | aVarTruthTableCondition_5 = logical(bmlID==5);
    | 
    | 
    | aVarTruthTableCondition_6 = logical(bmlID==6);
    | 
    | 
    | aVarTruthTableCondition_7 = logical(bmlID==7);
    | 
    | 
    | aVarTruthTableCondition_8 = logical(bmlID==8);
    | 
    | 
    | aVarTruthTableCondition_9 = logical(bmlID==9);
    | 
    | 
    | aVarTruthTableCondition_10 = logical(bmlID==10);
    | 
    | 
    | aVarTruthTableCondition_11 = logical(bmlID==11);
    | 
    | 
    | aVarTruthTableCondition_12 = logical(bmlID==12);
    | 
    | if (aVarTruthTableCondition_1)
    |     aFcnTruthTableAction_1();
    | elseif (aVarTruthTableCondition_2)
    |     aFcnTruthTableAction_2();
    | elseif (aVarTruthTableCondition_3)
    |     aFcnTruthTableAction_3();
    | elseif (aVarTruthTableCondition_4)
    |     aFcnTruthTableAction_4();
    | elseif (aVarTruthTableCondition_5)
    |     aFcnTruthTableAction_5();
    | elseif (aVarTruthTableCondition_6)
    |     aFcnTruthTableAction_6();
    | elseif (aVarTruthTableCondition_7)
    |     aFcnTruthTableAction_7();
    | elseif (aVarTruthTableCondition_8)
    |     aFcnTruthTableAction_8();
    | elseif (aVarTruthTableCondition_9)
    |     aFcnTruthTableAction_9();
    | elseif (aVarTruthTableCondition_10)
    |     aFcnTruthTableAction_10();
    | elseif (aVarTruthTableCondition_11)
    |     aFcnTruthTableAction_11();
    | elseif (aVarTruthTableCondition_12)
    |     aFcnTruthTableAction_12();
    | else % Default
    |     aFcnTruthTableAction_7();
    | end
    | 
    | function aFcnTruthTableAction_1()
    | 
    | % UpLeft
    | 
    | gazeBML=encStr2Arr('<?xml version="1.0" ?><act><bml><gaze angle="10" direction="UPLEFT" sbm:joint-range="EYES NECK" sbm:time-hint="1" target="gazeTarget"/></bml></act>');p=3;
    | 
    | function aFcnTruthTableAction_2()
    | 
    | % UpRight
    | 
    | gazeBML=encStr2Arr('<?xml version="1.0" ?><act><bml><gaze angle="10" direction="UPRIGHT" sbm:joint-range="EYES NECK" sbm:time-hint="1" target="gazeTarget"/></bml></act>');p=3;
    | 
    | function aFcnTruthTableAction_3()
    | 
    | % DownLeft
    | 
    | gazeBML=encStr2Arr('<?xml version="1.0" ?><act><bml><gaze angle="10" direction="DOWNLEFT" sbm:joint-range="EYES NECK" sbm:time-hint="1" target="gazeTarget"/></bml></act>');p=3;
    | 
    | function aFcnTruthTableAction_4()
    | 
    | % DownRight
    | 
    | gazeBML=encStr2Arr('<?xml version="1.0" ?><act><bml><gaze angle="10" direction="DOWNRIGHT" sbm:joint-range="EYES NECK" sbm:time-hint="1" target="gazeTarget"/></bml></act>');p=3;
    | 
    | function aFcnTruthTableAction_5()
    | 
    | % Down
    | 
    | gazeBML=encStr2Arr('<?xml version="1.0" ?><act><bml><gaze angle="10" direction="DOWN" sbm:joint-range="EYES NECK" sbm:time-hint="1" target="gazeTarget"/></bml></act>');p=3;
    | 
    | function aFcnTruthTableAction_6()
    | 
    | % Up
    | 
    | gazeBML=encStr2Arr('<?xml version="1.0" ?><act><bml><gaze direction="UP" angle="10" sbm:joint-range="EYES NECK" sbm:time-hint="1" target="gazeTarget"/></bml></act>');p=3;
    | 
    | function aFcnTruthTableAction_7()
    | 
    | % Right
    | 
    | gazeBML=encStr2Arr('<?xml version="1.0" ?><act><bml><gaze direction="RIGHT" angle="15" sbm:joint-range="EYES NECK" sbm:time-hint="1" target="gazeTarget"/></bml></act>');p=3;
    | 
    | function aFcnTruthTableAction_8()
    | 
    | % Left
    | 
    | gazeBML=encStr2Arr('<?xml version="1.0" ?><act><bml><gaze direction="LEFT" angle="15" sbm:joint-range="EYES NECK" sbm:time-hint="1" target="gazeTarget"/></bml></act>');p=3;
    | 
    | function aFcnTruthTableAction_9()
    | 
    | % RightS
    | 
    | gazeBML=encStr2Arr('<?xml version="1.0" ?><act><bml><gaze direction="RIGHT" angle="10" sbm:joint-range="EYES NECK" sbm:time-hint="1" target="gazeTarget"/></bml></act>');p=3;
    | 
    | function aFcnTruthTableAction_10()
    | 
    | % LeftS
    | 
    | gazeBML=encStr2Arr('<?xml version="1.0" ?><act><bml><gaze direction="LEFT" angle="10" sbm:joint-range="EYES NECK" sbm:time-hint="1" target="gazeTarget"/></bml></act>');p=3;
    | 
    | function aFcnTruthTableAction_11()
    | 
    | % neutralEye
    | 
    | gazeBML=encStr2Arr('<?xml version="1.0" ?><act><bml><gaze sbm:joint-range="EYES" target="gazeTarget"/></bml></act>'); p=3;
    | 
    | function aFcnTruthTableAction_12()
    | 
    | % neutralHead
    | 
    | gazeBML=encStr2Arr('<?xml version="1.0" ?><act><bml><gaze sbm:joint-range="EYES BACK" sbm:time-hint="1" target="gazeTarget"/></bml></act>'); p=3;
  function [p,gazeBML]=idleFastUpHeadTable(bmlID):
    | function [p,gazeBML]=idleFastUpHeadTable(bmlID)
    | 
    | aVarTruthTableCondition_1 = false;
    | aVarTruthTableCondition_2 = false;
    | aVarTruthTableCondition_3 = false;
    | aVarTruthTableCondition_4 = false;
    | aVarTruthTableCondition_5 = false;
    | aVarTruthTableCondition_6 = false;
    | aVarTruthTableCondition_7 = false;
    | aVarTruthTableCondition_8 = false;
    | aVarTruthTableCondition_9 = false;
    | aVarTruthTableCondition_10 = false;
    | aVarTruthTableCondition_11 = false;
    | aVarTruthTableCondition_12 = false;
    | aVarTruthTableCondition_13 = false;
    | aVarTruthTableCondition_14 = false;
    | aVarTruthTableCondition_15 = false;
    | aVarTruthTableCondition_16 = false;
    | aVarTruthTableCondition_17 = false;
    | aVarTruthTableCondition_18 = false;
    | aVarTruthTableCondition_19 = false;
    | aVarTruthTableCondition_20 = false;
    | aVarTruthTableCondition_21 = false;
    | aVarTruthTableCondition_22 = false;
    | 
    | 
    | 
    | aVarTruthTableCondition_1 = logical(bmlID==1);
    | 
    | 
    | aVarTruthTableCondition_2 = logical(bmlID==2);
    | 
    | 
    | aVarTruthTableCondition_3 = logical(bmlID==3);
    | 
    | 
    | aVarTruthTableCondition_4 = logical(bmlID==4);
    | 
    | 
    | aVarTruthTableCondition_5 = logical(bmlID==5);
    | 
    | 
    | aVarTruthTableCondition_6 = logical(bmlID==6);
    | 
    | 
    | aVarTruthTableCondition_7 = logical(bmlID==7);
    | 
    | 
    | aVarTruthTableCondition_8 = logical(bmlID==8);
    | 
    | 
    | aVarTruthTableCondition_9 = logical(bmlID==9);
    | 
    | 
    | aVarTruthTableCondition_10 = logical(bmlID==10);
    | 
    | 
    | aVarTruthTableCondition_11 = logical(bmlID==11);
    | 
    | 
    | aVarTruthTableCondition_12 = logical(bmlID==12);
    | 
    | 
    | aVarTruthTableCondition_13 = logical(bmlID==13);
    | 
    | 
    | aVarTruthTableCondition_14 = logical(bmlID==14);
    | 
    | 
    | aVarTruthTableCondition_15 = logical(bmlID==15);
    | 
    | 
    | aVarTruthTableCondition_16 = logical(bmlID==16);
    | 
    | 
    | aVarTruthTableCondition_17 = logical(bmlID==17);
    | 
    | 
    | aVarTruthTableCondition_18 = logical(bmlID==18);
    | 
    | 
    | aVarTruthTableCondition_19 = logical(bmlID==19);
    | 
    | 
    | aVarTruthTableCondition_20 = logical(bmlID==20);
    | 
    | 
    | aVarTruthTableCondition_21 = logical(bmlID==21);
    | 
    | 
    | aVarTruthTableCondition_22 = logical(bmlID==22);
    | 
    | if (aVarTruthTableCondition_1)
    |     aFcnTruthTableAction_1();
    | elseif (aVarTruthTableCondition_2)
    |     aFcnTruthTableAction_2();
    | elseif (aVarTruthTableCondition_3)
    |     aFcnTruthTableAction_3();
    | elseif (aVarTruthTableCondition_4)
    |     aFcnTruthTableAction_4();
    | elseif (aVarTruthTableCondition_5)
    |     aFcnTruthTableAction_5();
    | elseif (aVarTruthTableCondition_6)
    |     aFcnTruthTableAction_6();
    | elseif (aVarTruthTableCondition_7)
    |     aFcnTruthTableAction_7();
    | elseif (aVarTruthTableCondition_8)
    |     aFcnTruthTableAction_8();
    | elseif (aVarTruthTableCondition_9)
    |     aFcnTruthTableAction_9();
    | elseif (aVarTruthTableCondition_10)
    |     aFcnTruthTableAction_10();
    | elseif (aVarTruthTableCondition_11)
    |     aFcnTruthTableAction_11();
    | elseif (aVarTruthTableCondition_12)
    |     aFcnTruthTableAction_12();
    | elseif (aVarTruthTableCondition_13)
    |     aFcnTruthTableAction_13();
    | elseif (aVarTruthTableCondition_14)
    |     aFcnTruthTableAction_14();
    | elseif (aVarTruthTableCondition_15)
    |     aFcnTruthTableAction_15();
    | elseif (aVarTruthTableCondition_16)
    |     aFcnTruthTableAction_16();
    | elseif (aVarTruthTableCondition_17)
    |     aFcnTruthTableAction_17();
    | elseif (aVarTruthTableCondition_18)
    |     aFcnTruthTableAction_18();
    | elseif (aVarTruthTableCondition_19)
    |     aFcnTruthTableAction_19();
    | elseif (aVarTruthTableCondition_20)
    |     aFcnTruthTableAction_20();
    | elseif (aVarTruthTableCondition_21)
    |     aFcnTruthTableAction_21();
    | elseif (aVarTruthTableCondition_22)
    |     aFcnTruthTableAction_22();
    | else % Default
    |     aFcnTruthTableAction_1();
    | end
    | 
    | function aFcnTruthTableAction_1()
    | 
    | % UprightHead1
    | 
    | gazeBML=encStr2Arr('<?xml version="1.0" ?><act><bml><gaze direction="UPRIGHT" angle="15" sbm:joint-range="EYES NECK" target="gazeTarget"/></bml></act>');p=3;
    | 
    | function aFcnTruthTableAction_2()
    | 
    | % UprightHead2
    | 
    | gazeBML=encStr2Arr('<?xml version="1.0" ?><act><bml><gaze direction="UPRIGHT" angle="20" sbm:joint-range="EYES NECK" target="gazeTarget"/></bml></act>');p=3;
    | 
    | function aFcnTruthTableAction_3()
    | 
    | % UprightHead3
    | 
    | gazeBML=encStr2Arr('<?xml version="1.0" ?><act><bml><gaze direction="UPRIGHT" angle="25" sbm:joint-range="EYES NECK" target="gazeTarget"/></bml></act>');p=3;
    | 
    | function aFcnTruthTableAction_4()
    | 
    | % UprightHead4
    | 
    | gazeBML=encStr2Arr('<?xml version="1.0" ?><act><bml><gaze direction="UPRIGHT" angle="30" sbm:joint-range="EYES NECK" target="gazeTarget"/></bml></act>');p=3;
    | 
    | function aFcnTruthTableAction_5()
    | 
    | % UpleftHead1
    | 
    | gazeBML=encStr2Arr('<?xml version="1.0" ?><act><bml><gaze direction="UPLEFT" angle="15" sbm:joint-range="EYES NECK" target="gazeTarget"/></bml></act>');p=3;
    | 
    | function aFcnTruthTableAction_6()
    | 
    | % UpleftHead2
    | 
    | gazeBML=encStr2Arr('<?xml version="1.0" ?><act><bml><gaze direction="UPLEFT" angle="20" sbm:joint-range="EYES NECK"  target="gazeTarget"/></bml></act>');p=3;
    | 
    | function aFcnTruthTableAction_7()
    | 
    | % UpleftHead3
    | 
    | gazeBML=encStr2Arr('<?xml version="1.0" ?><act><bml><gaze direction="UPLEFT" angle="25" sbm:joint-range="EYES NECK"  target="gazeTarget"/></bml></act>');p=3;
    | 
    | function aFcnTruthTableAction_8()
    | 
    | % UpleftHead4
    | 
    | gazeBML=encStr2Arr('<?xml version="1.0" ?><act><bml><gaze direction="UPLEFT" angle="30" sbm:joint-range="EYES NECK"  target="gazeTarget"/></bml></act>');p=3;
    | 
    | function aFcnTruthTableAction_9()
    | 
    | % UpHead1
    | 
    | gazeBML=encStr2Arr('<?xml version="1.0" ?><act><bml><gaze direction="UP" angle="12" sbm:joint-range="EYES NECK"  target="gazeTarget"/><gaze angle="10" direction="UP" sbm:joint-range="EYES" target="camera"/></bml></act>');p=3;
    | 
    | function aFcnTruthTableAction_10()
    | 
    | % UpHead2
    | 
    | gazeBML=encStr2Arr('<?xml version="1.0" ?><act><bml><gaze direction="UP" angle="15" sbm:joint-range="EYES NECK" target="gazeTarget"/><gaze angle="10" direction="UP" sbm:joint-range="EYES" target="camera"/></bml></act>');p=3;
    | 
    | function aFcnTruthTableAction_11()
    | 
    | % RightHead1
    | 
    | gazeBML=encStr2Arr('<?xml version="1.0" ?><act><bml><gaze direction="RIGHT" angle="10" sbm:joint-range="EYES NECK"  target="gazeTarget"/></bml></act>');p=3;
    | 
    | function aFcnTruthTableAction_12()
    | 
    | % RightHead2
    | 
    | gazeBML=encStr2Arr('<?xml version="1.0" ?><act><bml><gaze direction="RIGHT" angle="15" sbm:joint-range="EYES NECK"  target="gazeTarget"/></bml></act>');p=3;
    | 
    | function aFcnTruthTableAction_13()
    | 
    | % RightHead3
    | 
    | gazeBML=encStr2Arr('<?xml version="1.0" ?><act><bml><gaze direction="RIGHT" angle="20" sbm:joint-range="EYES NECK"  target="gazeTarget"/></bml></act>');p=3;
    | 
    | function aFcnTruthTableAction_14()
    | 
    | % RightHead4
    | 
    | gazeBML=encStr2Arr('<?xml version="1.0" ?><act><bml><gaze direction="RIGHT" angle="25" sbm:joint-range="EYES NECK"  target="gazeTarget"/></bml></act>');p=3;
    | 
    | function aFcnTruthTableAction_15()
    | 
    | % RightHead5
    | 
    | gazeBML=encStr2Arr('<?xml version="1.0" ?><act><bml><gaze direction="RIGHT" angle="30" sbm:joint-range="EYES NECK"  target="gazeTarget"/></bml></act>');p=3;
    | 
    | function aFcnTruthTableAction_16()
    | 
    | % LEFTHead1
    | 
    | gazeBML=encStr2Arr('<?xml version="1.0" ?><act><bml><gaze direction="LEFT" angle="10" sbm:joint-range="EYES NECK"  target="gazeTarget"/></bml></act>');p=3;
    | 
    | function aFcnTruthTableAction_17()
    | 
    | % LEFTHead2
    | 
    | gazeBML=encStr2Arr('<?xml version="1.0" ?><act><bml><gaze direction="LEFT" angle="15" sbm:joint-range="EYES NECK"  target="gazeTarget"/></bml></act>');p=3;
    | 
    | function aFcnTruthTableAction_18()
    | 
    | % LEFTHead3
    | 
    | gazeBML=encStr2Arr('<?xml version="1.0" ?><act><bml><gaze direction="LEFT" angle="20" sbm:joint-range="EYES NECK"  target="gazeTarget"/></bml></act>');p=3;
    | 
    | function aFcnTruthTableAction_19()
    | 
    | % LEFTHead4
    | 
    | gazeBML=encStr2Arr('<?xml version="1.0" ?><act><bml><gaze direction="LEFT" angle="25" sbm:joint-range="EYES NECK"  target="gazeTarget"/></bml></act>');p=3;
    | 
    | function aFcnTruthTableAction_20()
    | 
    | % LEFTHead5
    | 
    | gazeBML=encStr2Arr('<?xml version="1.0" ?><act><bml><gaze direction="LEFT" angle="30" sbm:joint-range="EYES NECK"  target="gazeTarget"/></bml></act>');p=3;
    | 
    | function aFcnTruthTableAction_21()
    | 
    | % neutralEyeExtrovert
    | 
    | gazeBML=encStr2Arr('<?xml version="1.0" ?><act><bml><gaze sbm:joint-range="EYES" target="gazeTarget"/></bml></act>'); p=3;
    | 
    | function aFcnTruthTableAction_22()
    | 
    | % neutralHeadExtrovert
    | 
    | gazeBML=encStr2Arr('<?xml version="1.0" ?><act><bml><gaze angle="5" direction="UP" sbm:joint-range="EYES BACK" target="gazeTarget"/></bml></act>'); p=3;
  function [p,gazeBML]=gazeFollowUserMove(bmlID):
    | function [p,gazeBML]=gazeFollowUserMove(bmlID)
    | 
    | aVarTruthTableCondition_1 = false;
    | aVarTruthTableCondition_2 = false;
    | aVarTruthTableCondition_3 = false;
    | 
    | 
    | % r
    | 
    | aVarTruthTableCondition_1 = logical(bmlID==1);
    | 
    | % l
    | 
    | aVarTruthTableCondition_2 = logical(bmlID==2);
    | 
    | % n
    | 
    | aVarTruthTableCondition_3 = logical(bmlID==3);
    | 
    | if (aVarTruthTableCondition_1)
    |     aFcnTruthTableAction_1();
    | elseif (aVarTruthTableCondition_2)
    |     aFcnTruthTableAction_2();
    | elseif (aVarTruthTableCondition_3)
    |     aFcnTruthTableAction_3();
    | else % Default
    |     aFcnTruthTableAction_3();
    | end
    | 
    | function aFcnTruthTableAction_1()
    | 
    | % gazeRight
    | 
    | gazeBML=encStr2Arr( '<?xml version="1.0" ?><act><bml><gaze angle="7" direction="RIGHT" sbm:joint-range="HEAD BACK" sbm:time-hint="1.5" target="gazeTarget"/></bml></act>');p=1;
    | 
    | function aFcnTruthTableAction_2()
    | 
    | % gazeLeft
    | 
    | gazeBML=encStr2Arr( '<?xml version="1.0" ?><act><bml><gaze angle="12" direction="LEFT" sbm:joint-range="HEAD BACK" sbm:time-hint="1.5" target="gazeTarget"/></bml></act>');p=1;
    | 
    | function aFcnTruthTableAction_3()
    | 
    | % neutral
    | 
    | gazeBML=encStr2Arr( '<?xml version="1.0" ?><act><bml><gaze sbm:time-hint="1.5" target="gazeTarget"/></bml></act>');p=1;
  function [p,gazeBML]=idleGazeInterestedTable(bmlID):
    | function [p,gazeBML]=idleGazeInterestedTable(bmlID)
    | 
    | aVarTruthTableCondition_1 = false;
    | aVarTruthTableCondition_2 = false;
    | aVarTruthTableCondition_3 = false;
    | aVarTruthTableCondition_4 = false;
    | aVarTruthTableCondition_5 = false;
    | aVarTruthTableCondition_6 = false;
    | aVarTruthTableCondition_7 = false;
    | aVarTruthTableCondition_8 = false;
    | 
    | 
    | 
    | aVarTruthTableCondition_1 = logical(bmlID==1);
    | 
    | 
    | aVarTruthTableCondition_2 = logical(bmlID==2);
    | 
    | 
    | aVarTruthTableCondition_3 = logical(bmlID==3);
    | 
    | 
    | aVarTruthTableCondition_4 = logical(bmlID==4);
    | 
    | 
    | aVarTruthTableCondition_5 = logical(bmlID==5);
    | 
    | 
    | aVarTruthTableCondition_6 = logical(bmlID==6);
    | 
    | 
    | aVarTruthTableCondition_7 = logical(bmlID==7);
    | 
    | 
    | aVarTruthTableCondition_8 = logical(bmlID==8);
    | 
    | if (aVarTruthTableCondition_1)
    |     aFcnTruthTableAction_1();
    | elseif (aVarTruthTableCondition_2)
    |     aFcnTruthTableAction_2();
    | elseif (aVarTruthTableCondition_3)
    |     aFcnTruthTableAction_3();
    | elseif (aVarTruthTableCondition_4)
    |     aFcnTruthTableAction_4();
    | elseif (aVarTruthTableCondition_5)
    |     aFcnTruthTableAction_5();
    | elseif (aVarTruthTableCondition_6)
    |     aFcnTruthTableAction_6();
    | elseif (aVarTruthTableCondition_7)
    |     aFcnTruthTableAction_7();
    | elseif (aVarTruthTableCondition_8)
    |     aFcnTruthTableAction_8();
    | else % Default
    |     aFcnTruthTableAction_1();
    | end
    | 
    | function aFcnTruthTableAction_1()
    | 
    | % UpS
    | 
    | gazeBML=encStr2Arr('<?xml version="1.0" ?><act><bml><gaze angle="5" direction="UP" sbm:joint-range="EYES" target="camera"/></bml></act>');p=3;
    | 
    | function aFcnTruthTableAction_2()
    | 
    | % DownS
    | 
    | gazeBML=encStr2Arr('<?xml version="1.0" ?><act><bml><gaze angle="5" direction="DOWN" sbm:joint-range="EYES" target="camera"/></bml></act>');p=3;
    | 
    | function aFcnTruthTableAction_3()
    | 
    | % DownS
    | 
    | gazeBML=encStr2Arr('<?xml version="1.0" ?><act><bml><gaze angle="10" direction="DOWN" sbm:joint-range="EYES" target="camera"/></bml></act>');p=3;
    | 
    | function aFcnTruthTableAction_4()
    | 
    | % UpLeft3
    | 
    | gazeBML=encStr2Arr('<?xml version="1.0" ?><act><bml><gaze angle="3" direction="UPLEFT" sbm:joint-range="EYES" target="camera"/></bml></act>');p=3;
    | 
    | function aFcnTruthTableAction_5()
    | 
    | % UpRight3
    | 
    | gazeBML=encStr2Arr('<?xml version="1.0" ?><act><bml><gaze angle="3" direction="UPRIGHT" sbm:joint-range="EYES" target="camera"/></bml></act>');p=3;
    | 
    | function aFcnTruthTableAction_6()
    | 
    | % DownLeft3
    | 
    | gazeBML=encStr2Arr('<?xml version="1.0" ?><act><bml><gaze angle="3" direction="DOWNLEFT" sbm:joint-range="EYES" target="camera"/></bml></act>');p=3;
    | 
    | function aFcnTruthTableAction_7()
    | 
    | % DownRight3
    | 
    | gazeBML=encStr2Arr('<?xml version="1.0" ?><act><bml><gaze angle="3" direction="DOWNRIGHT" sbm:joint-range="EYES" target="camera"/></bml></act>');p=3;
    | 
    | function aFcnTruthTableAction_8()
    | 
    | % UpPolar10
    | 
    | gazeBML=encStr2Arr('<?xml version="1.0" ?><act><bml><gaze angle="10" direction="POLAR" sbm:joint-range="EYES" sbm:time-hint="1.5" target="camera"/></bml></act>');p=3;
  function arrBML    = idleGazeOrigFunction(dir,mag):
    | function arrBML    = idleGazeOrigFunction(dir,mag)
    | coder.extrinsic('sprintf') 
    | %8 percent chance of not pure(UR,UL,DR,DL) and 25 percent chance of pure
    | %angle(U,D,L,R)
    |  if (0<dir)&&(dir<=24)
    |      dirG='UP';
    |      cDir=2;
    |  elseif (25<dir)&&(dir<=49)
    |      dirG='DOWN';
    |      cDir=4;
    |  elseif (50<dir)&&(dir<=74)
    |      dirG='RIGHT';
    |      cDir=5;
    |  elseif (75<dir)&&(dir<=99)
    |      dirG='LEFT';
    |      cDir=4;
    |  elseif (100<dir)&&(dir<=107)
    |      dirG='UPRIGHT';
    |      cDir=7;
    |  elseif (108<dir)&&(dir<=115) 
    |      dirG='UPLEFT';
    |      cDir=6;
    |  elseif (116<dir)&&(dir<=124)
    |      dirG='DOWNRIGHT';
    |      cDir=9;
    |  elseif (125<dir)&&(dir<=132)
    |      dirG='DOWNLEFT';
    |      cDir=8;
    |  else
    |      dirG='LEFT';
    |      cDir=4;
    |  end
    |  c = countDigits(mag);
    | 
    |  mystr=blanks(125+c+cDir); %btw 2 and 9 for dirG , for m btw 1 and 2
    |  mystr  = sprintf('<?xml version="1.0" ?><act><bml><gaze angle="%d" direction="%s" sbm:joint-range="EYES" target="gazeTarget"/></bml></act>',mag,dirG);
    |  arrBML = encStr2Arr(mystr);
  function [p,poseBML] = successTable(bmlID):
    | function [p,poseBML] = successTable(bmlID)
    | 
    | aVarTruthTableCondition_1 = false;
    | aVarTruthTableCondition_2 = false;
    | aVarTruthTableCondition_3 = false;
    | 
    | 
    | % smile
    | 
    | aVarTruthTableCondition_1 = logical(bmlID==1);
    | 
    | % HeadChestUp
    | 
    | aVarTruthTableCondition_2 = logical(bmlID==2);
    | 
    | % browUp
    | 
    | aVarTruthTableCondition_3 = logical(bmlID==3);
    | 
    | if (aVarTruthTableCondition_1)
    |     aFcnTruthTableAction_1();
    | elseif (aVarTruthTableCondition_2)
    |     aFcnTruthTableAction_2();
    | elseif (aVarTruthTableCondition_3)
    |     aFcnTruthTableAction_3();
    | else % Default
    |     aFcnTruthTableAction_1();
    | end
    | 
    | function aFcnTruthTableAction_1()
    | 
    | % smile
    | 
    | poseBML=encStr2Arr('<?xml version="1.0" ?><act><bml><face amount="1" side="BOTH" au="12" start="0" stroke="4" relax="8" end="10"  type="facs"/><face amount="0.5" au="6" side="BOTH" start="0" stroke="4" stroke="3" relax="8" end="15" type="facs"/></bml></act>');p=3;
    | 
    | function aFcnTruthTableAction_2()
    | 
    | % HeadChestUp
    | 
    | poseBML=encStr2Arr('<?xml version="1.0" ?><act><bml><gaze angle="12" direction="UP" sbm:joint-range="HEAD CHEST" sbm:time-hint="1.5" target="camera"/></bml></act>');p=3;
    | 
    | function aFcnTruthTableAction_3()
    | 
    | % browUp
    | 
    | poseBML=encStr2Arr('<?xml version="1.0" ?><act><bml><face amount="0.3" au="1" side="BOTH" start="0" end="15" type="facs"/><face amount="0.3"  au="2" end="15" side="BOTH" start="0" type="facs"/></bml></act>');p=3;
  function arrBML    = idleHeadFunction(dir,mag,dirChance,headSpeed):
    | function arrBML    = idleHeadFunction(dir,mag,dirChance,headSpeed)
    | coder.extrinsic('sprintf') 
    | %total: 132 is 8 percent chance of not pure(UR,UL,DR,DL) and 25 percent chance of pure(U,D,L,R)
    | %for extroverts low chance of look down: 131 is
    |                   %2 percent chance of not pure down(DR,DL) 
    |                   %14 percent chance of  each of other not pures(UR,UL)
    |                   %6 percent chance of pure down(D)
    |                   %31 percent chance of each of other pures(U,L,R)
    | %for introverts low chance of look up: 131 is
    |                   %2 percent chance of not pure up(UR,UL) 
    |                   %14 percent chance of  each of other not pures(DR,DL)
    |                   %6 percent chance of pure up(U)
    |                   %64 percent chance of down, %15 each of other pures(L,R)
    | if(dirChance==1) %extrovert: HEHN,HELN, Switched Up and Upright since UP does not look good
    |     if (0<dir)&&(dir<=31) %  %31 U, L & R, 6% D ; 
    |          dirG='UPRIGHT';
    |          cDir=7;
    |      elseif (31<dir)&&(dir<=35)
    |          dirG='DOWN';
    |          cDir=4;
    |      elseif (35<dir)&&(dir<=67)
    |          dirG='RIGHT';
    |          cDir=5;
    |      elseif (67<dir)&&(dir<=99)
    |          dirG='LEFT';
    |          cDir=4;
    |           %14 UL&UR, %2 DL,DR
    |      elseif (99<dir)&&(dir<=113)
    |          dirG='UP';
    |          mag=mag-2;
    |          cDir=2;
    |      elseif (113<dir)&&(dir<=127) 
    |          dirG='UPLEFT';
    |          cDir=6;
    |      elseif (127<dir)&&(dir<=129)
    |          dirG='DOWNRIGHT';
    |          cDir=9;
    |      elseif (129<dir)&&(dir<=132)
    |          dirG='DOWNLEFT';
    |          cDir=8;
    |      else
    |          dirG='LEFT';
    |          cDir=4;
    |      end
    | elseif(dirChance==2)%introvert  6% U, 64% D, %15 L & R
    |      if (0<dir)&&(dir<=68)
    |          dirG='DOWN';
    |          cDir=4;
    |      elseif (68<dir)&&(dir<=70)
    |          dirG='UP';
    |          mag=mag-2;
    |          cDir=2;
    |      elseif (70<dir)&&(dir<=75)
    |          dirG='RIGHT';
    |          cDir=5;
    |      elseif (75<dir)&&(dir<=80)
    |          dirG='LEFT';
    |          cDir=4;
    |          %2 UL&UR, %14 DL,DR
    |      elseif (80<dir)&&(dir<=85)
    |          dirG='UPRIGHT';
    |          cDir=7;
    |      elseif (85<dir)&&(dir<=87) 
    |          dirG='UPLEFT';
    |          cDir=6;
    |      elseif (87<dir)&&(dir<=110)
    |          dirG='DOWNRIGHT';
    |          cDir=9;
    |      elseif (110<dir)&&(dir<=132)
    |          dirG='DOWNLEFT';
    |          cDir=8;
    |      else
    |          disp('gaze else');
    |          dirG='LEFT';
    |          cDir=4;
    |      end
    | else
    |     %8 percent chance of not pure(UR,UL,DR,DL) and 25 percent chance of pure
    |     %angle(U,D,L,R)
    |      if (0<dir)&&(dir<=24)
    |          dirG='UP';
    |          cDir=2;
    |      elseif (25<dir)&&(dir<=49)
    |          dirG='DOWN';
    |          cDir=4;
    |      elseif (50<dir)&&(dir<=74)
    |          dirG='RIGHT';
    |          cDir=5;
    |      elseif (75<dir)&&(dir<=99)
    |          dirG='LEFT';
    |          cDir=4;
    |      elseif (100<dir)&&(dir<=107)
    |          dirG='UPRIGHT';
    |          cDir=7;
    |      elseif (108<dir)&&(dir<=115) 
    |          dirG='UPLEFT';
    |          cDir=6;
    |      elseif (116<dir)&&(dir<=124)
    |          dirG='DOWNRIGHT';
    |          cDir=9;
    |      elseif (125<dir)&&(dir<=132)
    |          dirG='DOWNLEFT';
    |          cDir=8;
    |      else
    |          dirG='LEFT';
    |          cDir=4;   
    |      end
    | end
    |  c = countDigits(mag);
    | 
    |  %PROBLEM: rotate head to a random generated angle=this way? or fixed angles=old way
    | % fastupleft
    | % gazeBML=encStr2Arr('<?xml version="1.0" ?><act><bml><gaze direction="UPLEFT" angle="20" sbm:joint-range="EYES NECK" sbm:time-hint="1" target="gazeTarget"/></bml></act>');p=3;
    | % slowDown
    | % gazeBML=encStr2Arr('<?xml version="1.0" ?><act><bml><gaze direction="DOWN" angle="15" sbm:joint-range="EYES NECK" sbm:time-hint="1.2" target="gazeTarget"/></bml></act>');p=3;
    | 
    |  mystr=blanks(125+c+cDir); %btw 2 and 9 for dirG , for m btw 1 and 2
    |  mystr  = sprintf('<?xml version="1.0" ?><act><bml><gaze angle="%d" direction="%s" sbm:joint-range="EYES NECK" target="gazeTarget"/></bml></act>',mag,dirG);
    |  arrBML = encStr2Arr(mystr);
  function arrBML    = idleGazeFunction(dir,mag,dirChance):
    | function arrBML    = idleGazeFunction(dir,mag,dirChance)
    | coder.extrinsic('sprintf') 
    | %total: 132 is 8 percent chance of not pure(UR,UL,DR,DL) and 25 percent chance of pure(U,D,L,R)
    | %for extroverts low chance of look down: 131 is
    |                   %2 percent chance of not pure down(DR,DL) 
    |                   %14 percent chance of  each of other not pures(UR,UL)
    |                   %6 percent chance of pure down(D)
    |                   %31 percent chance of each of other pures(U,L,R)
    | %for introverts low chance of look up: 131 is
    |                   %2 percent chance of not pure up(UR,UL) 
    |                   %14 percent chance of  each of other not pures(DR,DL)
    |                   %6 percent chance of pure up(U)
    |                   %64 percent chance of down, %15 each of other pures(L,R)
    | if(dirChance==1) %extrovert: HEHN,HELN, Switched Up and Upright since UP does not look good
    |     if (0<dir)&&(dir<=31) %  %31 U, L & R, 6% D ; 
    |          dirG='UPRIGHT';
    |          cDir=7;
    |      elseif (31<dir)&&(dir<=35)
    |          dirG='DOWN';
    |          cDir=4;
    |      elseif (35<dir)&&(dir<=67)
    |          dirG='RIGHT';
    |          cDir=5;
    |      elseif (67<dir)&&(dir<=99)
    |          dirG='LEFT';
    |          cDir=4;
    |           %14 UL&UR, %2 DL,DR
    |      elseif (99<dir)&&(dir<=113)
    |          dirG='UP';
    |          mag=mag-2;
    |          cDir=2;
    |      elseif (113<dir)&&(dir<=127) 
    |          dirG='UPLEFT';
    |          cDir=6;
    |      elseif (127<dir)&&(dir<=129)
    |          dirG='DOWNRIGHT';
    |          cDir=9;
    |      elseif (129<dir)&&(dir<=132)
    |          dirG='DOWNLEFT';
    |          cDir=8;
    |      else
    |          dirG='LEFT';
    |          cDir=4;
    |      end
    | elseif(dirChance==2)%introvert  6% U, 64% D, %15 L & R
    |      if (0<dir)&&(dir<=68)
    |          dirG='DOWN';
    |          cDir=4;
    |      elseif (68<dir)&&(dir<=70)
    |          dirG='UP';
    |          mag=mag-2;
    |          cDir=2;
    |      elseif (70<dir)&&(dir<=75)
    |          dirG='RIGHT';
    |          cDir=5;
    |      elseif (75<dir)&&(dir<=80)
    |          dirG='LEFT';
    |          cDir=4;
    |          %2 UL&UR, %14 DL,DR
    |      elseif (80<dir)&&(dir<=85)
    |          dirG='UPRIGHT';
    |          cDir=7;
    |      elseif (85<dir)&&(dir<=87) 
    |          dirG='UPLEFT';
    |          cDir=6;
    |      elseif (87<dir)&&(dir<=110)
    |          dirG='DOWNRIGHT';
    |          cDir=9;
    |      elseif (110<dir)&&(dir<=132)
    |          dirG='DOWNLEFT';
    |          cDir=8;
    |      else
    |          disp('gaze else');
    |          dirG='LEFT';
    |          cDir=4;
    |      end
    | else
    |     %normal gaze
    |     %8 percent chance of not pure(UR,UL,DR,DL) and 25 percent chance of pure
    |     %angle(U,D,L,R)
    |      if (0<dir)&&(dir<=24)
    |          dirG='UP';
    |          cDir=2;
    |          mag=mag/2;
    |      elseif (25<dir)&&(dir<=49)
    |          dirG='DOWN';
    |          cDir=4;
    |      elseif (50<dir)&&(dir<=74)
    |          dirG='RIGHT';
    |          cDir=5;
    |      elseif (75<dir)&&(dir<=99)
    |          dirG='LEFT';
    |          cDir=4;
    |      elseif (100<dir)&&(dir<=107)
    |          dirG='UPRIGHT';
    |          cDir=7;
    |      elseif (108<dir)&&(dir<=115) 
    |          dirG='UPLEFT';
    |          cDir=6;
    |      elseif (116<dir)&&(dir<=124)
    |          dirG='DOWNRIGHT';
    |          cDir=9;
    |      elseif (125<dir)&&(dir<=132)
    |          dirG='DOWNLEFT';
    |          cDir=8;
    |      else
    |          dirG='LEFT';
    |          cDir=4;   
    |      end
    | end
    |  c = countDigits(mag);
    | 
    |  mystr=blanks(125+c+cDir); %btw 2 and 9 for dirG , for m btw 1 and 2
    |  mystr  = sprintf('<?xml version="1.0" ?><act><bml><gaze angle="%d" direction="%s" sbm:joint-range="EYES" target="gazeTarget"/></bml></act>',mag,dirG);
    |  arrBML = encStr2Arr(mystr);
  function newBmls =insertQueueLow(bmls,myBML):
    | function newBmls =insertQueueLow(bmls,myBML)
    |     full=1;
    |     t=encStr2Arr(' ');
    |     newBmls=[t t t t t];
    |     for i = 1:5
    |         if (isequal(bmls(:,i),t))
    |             %add to end of the queue where its empty
    |             bmls(:,i)=myBML;
    |             full=0;
    |             break
    |         end
    |     end
    |     if(full~=0)
    |             %if queue full, shift all elements to left which removes the first one, then add to end
    |             bmls(:,1)= bmls(:,2);
    |             bmls(:,2)= bmls(:,3);
    |             bmls(:,3)= bmls(:,4);
    |             bmls(:,5)=myBML;
    |     end
    |     newBmls=bmls;
  function arrSBM    = blinkFunction(blinkPeriodMin,blinkPeriodMax):
    | function arrSBM    = blinkFunction(blinkPeriodMin,blinkPeriodMax)
    |     coder.extrinsic('sprintf') 
    |     
    |     if(countDigits(blinkPeriodMax)> 1)
    |         mystr=blanks(168); 
    |     else
    |         mystr=blanks(167);
    |     end
    |     mystr  = sprintf(' mycharacter = scene.getCharacter("ChrBrad"); mycharacter.setDoubleAttribute("eyelid.blinkPeriodMin", %0.1f);mycharacter.setDoubleAttribute("eyelid.blinkPeriodMax", %0.1f)',blinkPeriodMin,blinkPeriodMax);
    |     arrSBM = encStr2Arr(mystr);
